simulink subsystem "robot_2021a"  (R2021a)
settings: Solver=VariableStepAuto  StartTime=0.0  StopTime=10.0  RelTol=1e-3
settings Model: Creator=marco  LastModifiedBy=marco

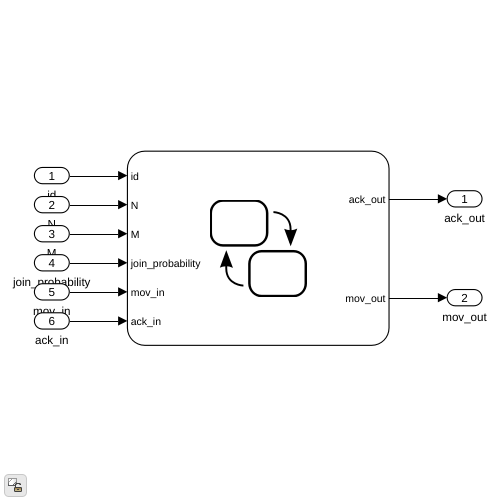
[thumbnail: Simulink's stored preview of the top-level diagram]
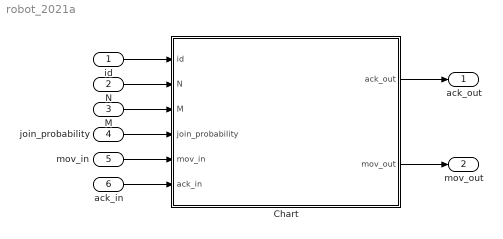
== system robot_2021a ==
  id : Inport
  N : Inport  Port=2
  M : Inport  Port=3
  join_probability : Inport  Port=4
  mov_in : Inport  Port=5
  ack_in : Inport  Port=6
  Chart : Stateflow chart  TreatAsAtomicUnit=on
  ack_out : Outport
  mov_out : Outport  Port=2
  wires:
  id/1 -> Chart/1(id)
  N/1 -> Chart/2(N)
  M/1 -> Chart/3(M)
  join_probability/1 -> Chart/4(join_probability)
  mov_in/1 -> Chart/5(mov_in)
  ack_in/1 -> Chart/6(ack_in)
  Chart/1(ack_out) -> ack_out/1
  Chart/2(mov_out) -> mov_out/1

== stateflow chart robot_2021a/Chart ==
  state Prepare
    entry:
    join = (join_probability > 0.3);
  state MovWait
    during:
    mov_out = -1;
    ack_out = ack_in;
  state AckWait
    entry:
    mov_out = pool_size;
    during:
    mov_out = -1;
  state CommonAction
    during:
    ack_out = 0;
    if (mov_in ~=- 1)
    ack_out = -1;
    end
  (default) -> MovWait : {first_node = (id == 0);
      | last_node = (id == N-1);}
  MovWait -> Prepare : [mov_in ~=- 1]{pool_size = mov_in;}
  Prepare -> (junction 69)
  CommonAction -> MovWait : % job done
      | after(2,sec)
  (junction 66) -> MovWait [order 2] : % middle node
      | {mov_out = pool_size}
  (junction 69) -> (junction 66) [order 2] : % not join
  (junction 66) -> (junction 77) [order 1] : [first_node || last_node]
  (junction 69) -> (junction 43) [order 1] : [join]{pool_size = pool_size + 1;}
  (junction 77) -> MovWait : {ack_out = -1;}
  (junction 43) -> (junction 59) [order 2] : % pool not formed
  (junction 59) -> (junction 77) [order 1] : [last_node]
  (junction 43) -> (junction 81) [order 1] : % pool formed
      | [pool_size == M]
  (junction 59) -> AckWait [order 2] : % middle node
  AckWait -> (junction 77) [order 2] : [ack_in == -1]
  AckWait -> (junction 81) [order 1] : [ack_in == 1]
  (junction 81) -> CommonAction : {ack_out = 1;}
  data: id input; N input; M input; join_probability input; ack_out output =0; mov_in input; mov_out output =-1; join local; pool_size local; ack_in input; last_node local; first_node local
